simulink model "ACC_2022b"  (R2022b)
settings: Solver=VariableStepAuto  StartTime=0.0  StopTime=inf  RelTol=1e-3
values from neighbouring files (symbols this model uses):
  b = 50    [ACC_code.m]
  D_default = 10    [ACC_code.m]
  m = 1000    [ACC_code.m]
undefined symbols (not defined in the file or in its folder): Ego_acceleration_max, Ego_acceleration_min, Ego_position_initial, Ego_velocity_initial_kmh, h, km, Kverr_gain, Kvx_gain, Kxerr_gain, Lead_position_initial, Lead_velocity_initial_kmh, s
libraries: aerolibconvert2 x6
settings Model: PacingRate=2  Creator=Leo  LastModifiedBy=Usuario
settings OptimizationCC: BlockReduction=off  DefaultParameterBehavior=Inlined  BufferReuse=off  ReuseModelBlockBuffer=on

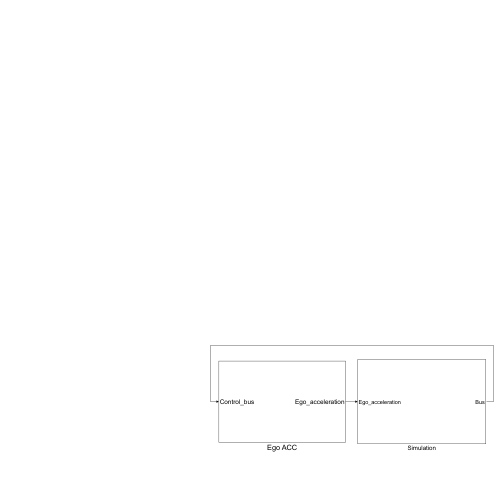
[thumbnail: Simulink's stored preview of the top-level diagram]
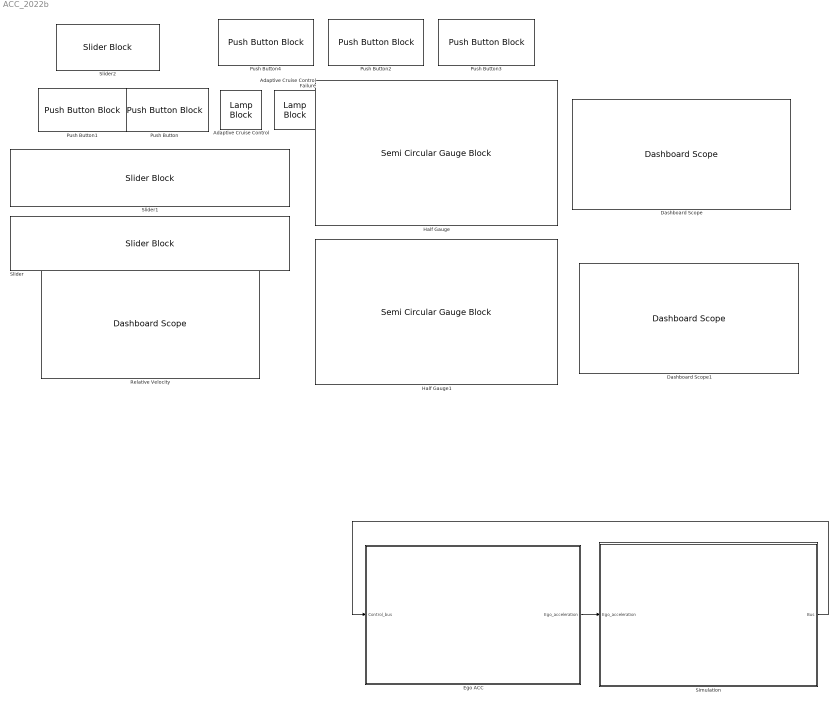
== system ACC_2022b ==
  Adaptive Cruise Control : LampBlock  LabelPosition=Hide  Icon=AdaptiveCruiseControl
  Adaptive Cruise Control Failure : LampBlock  LabelPosition=Hide  Icon=AdaptiveCruiseControlFailure
  Dashboard Scope : DashboardScope
  Dashboard Scope1 : DashboardScope
  Ego ACC : Subsystem
  Half Gauge : SemiCircularGaugeBlock  ScaleMax=220  TickInterval=20
  Half Gauge1 : SemiCircularGaugeBlock  ScaleMax=220  TickInterval=20
  Push Button : PushButtonBlock  ButtonText=ACC  OffValue=0.000000
  Push Button1 : PushButtonBlock  ButtonText=Rain  OffValue=0.000000
  Push Button2 : PushButtonBlock  ButtonText=Gas  ButtonType=Latch
  Push Button3 : PushButtonBlock  ButtonText=Brake  ButtonType=Latch
  Push Button4 : PushButtonBlock  ButtonText=Fault  ButtonType=Latch  OffValue=0.000000
  Relative Velocity : DashboardScope
  Simulation : Subsystem
  Slider : SliderBlock  ScaleMax=220  TickInterval=50
  Slider1 : SliderBlock  ScaleMin=40  ScaleMax=220  TickInterval=50
  Slider2 : SliderBlock  ScaleMin=1  ScaleMax=3  TickInterval=0.5
  wires:
  Ego ACC/1(Ego_acceleration) -> Simulation/1(Ego_acceleration)
  Simulation/1(Bus) -> Ego ACC/1(Control_bus)

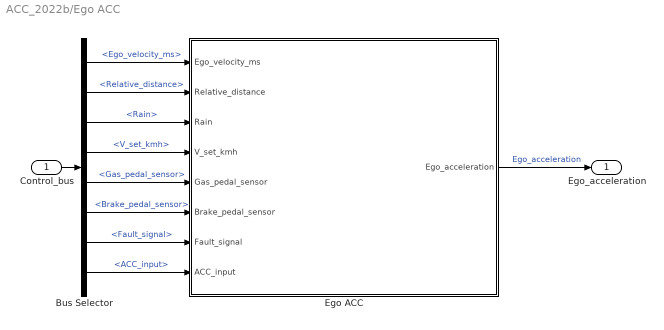
== system ACC_2022b/Ego ACC ==
  Control_bus : Inport
  Bus Selector : BusSelector  OutputSignals=Ego_velocity_ms,Relative_distance,Rain,V_set_kmh,Gas_pedal_sensor,Brake_pedal_sensor,Fault_signal,ACC_input
  Ego ACC : Subsystem
  Ego_acceleration : Outport
  wires:
  Control_bus/1 -> Bus Selector/1
  Ego ACC/1(Ego_acceleration) -> Ego_acceleration/1  "Ego_acceleration"
  Bus Selector/1 -> Ego ACC/1(Ego_velocity_ms)  "<Ego_velocity_ms>"
  Bus Selector/2 -> Ego ACC/2(Relative_distance)  "<Relative_distance>"
  Bus Selector/3 -> Ego ACC/3(Rain)  "<Rain>"
  Bus Selector/4 -> Ego ACC/4(V_set_kmh)  "<V_set_kmh>"
  Bus Selector/5 -> Ego ACC/5(Gas_pedal_sensor)  "<Gas_pedal_sensor>"
  Bus Selector/6 -> Ego ACC/6(Brake_pedal_sensor)  "<Brake_pedal_sensor>"
  Bus Selector/7 -> Ego ACC/7(Fault_signal)  "<Fault_signal>"
  Bus Selector/8 -> Ego ACC/8(ACC_input)  "<ACC_input>"

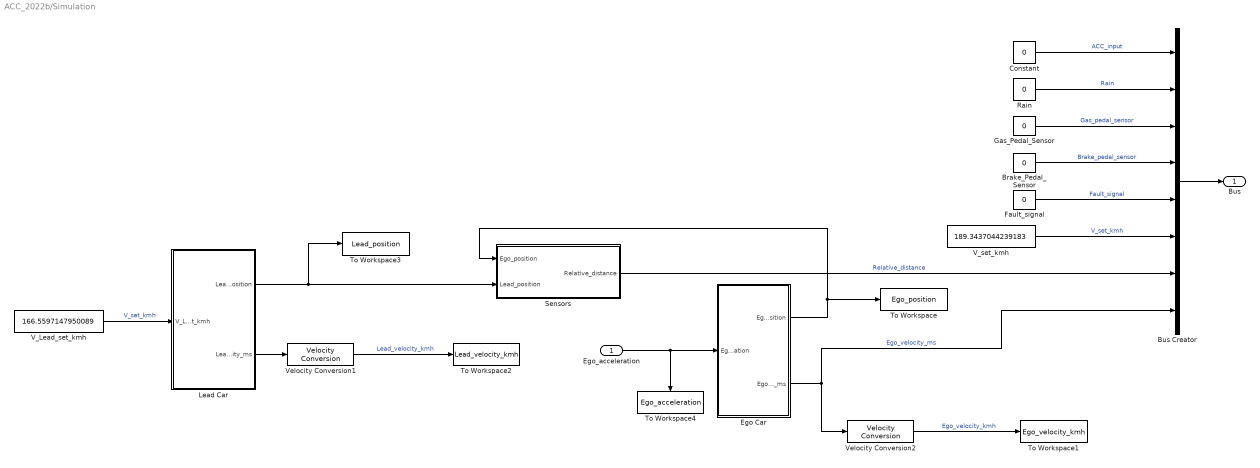
== system ACC_2022b/Simulation ==
  Ego_acceleration : Inport
  Brake_Pedal_Sensor : Constant  Value=0  SampleTime=-1
  Bus Creator : BusCreator  Inputs=8
  Constant : Constant  Value=0
  Ego Car : Subsystem
  Fault_signal : Constant  Value=0  SampleTime=-1
  Gas_Pedal_Sensor : Constant  Value=0  SampleTime=-1
  Lead Car : Subsystem
  Rain : Constant  Value=0
  Sensors : Subsystem
  To Workspace : ToWorkspace  VariableName=Ego_position  SaveFormat=Timeseries  SampleTime=-1
  To Workspace1 : ToWorkspace  VariableName=Ego_velocity_kmh  SaveFormat=Timeseries  SampleTime=-1
  To Workspace2 : ToWorkspace  VariableName=Lead_velocity_kmh  SaveFormat=Timeseries  SampleTime=-1
  To Workspace3 : ToWorkspace  VariableName=Lead_position  SaveFormat=Timeseries  SampleTime=-1
  To Workspace4 : ToWorkspace  VariableName=Ego_acceleration  SaveFormat=Timeseries  SampleTime=-1
  V_Lead_set_kmh : Constant  Value=166.5597147950089  SampleTime=-1
  V_set_kmh : Constant  Value=189.3437044239183  SampleTime=-1
  Velocity Conversion1 : aerolibconvert2/Velocity Conversion  IU=m/s  OU=km/h
  Velocity Conversion2 : aerolibconvert2/Velocity Conversion  IU=m/s  OU=km/h
  Bus : Outport
  wires:
  Constant/1 -> Bus Creator/1  "ACC_input"
  Lead Car/1(Lead_position) -> To Workspace3/1, Sensors/2(Lead_position)
  Fault_signal/1 -> Bus Creator/5  "Fault_signal"
  Sensors/1(Relative_distance) -> Bus Creator/7  "Relative_distance"
  Rain/1 -> Bus Creator/2  "Rain"
  Gas_Pedal_Sensor/1 -> Bus Creator/3  "Gas_pedal_sensor"
  Ego Car/1(Ego_position) -> To Workspace/1, Sensors/1(Ego_position)
  Brake_Pedal_Sensor/1 -> Bus Creator/4  "Brake_pedal_sensor"
  V_set_kmh/1 -> Bus Creator/6  "V_set_kmh"
  Ego Car/2(Ego_velocity_ms) -> Velocity Conversion2/1, Bus Creator/8  "Ego_velocity_ms"
  Bus Creator/1 -> Bus/1
  Ego_acceleration/1 -> To Workspace4/1, Ego Car/1(Ego_acceleration)
  Velocity Conversion1/1 -> To Workspace2/1  "Lead_velocity_kmh"
  Velocity Conversion2/1 -> To Workspace1/1  "Ego_velocity_kmh"
  Lead Car/2(Lead_velocity_ms) -> Velocity Conversion1/1
  V_Lead_set_kmh/1 -> Lead Car/1(V_Lead_Set_kmh)  "V_set_kmh"

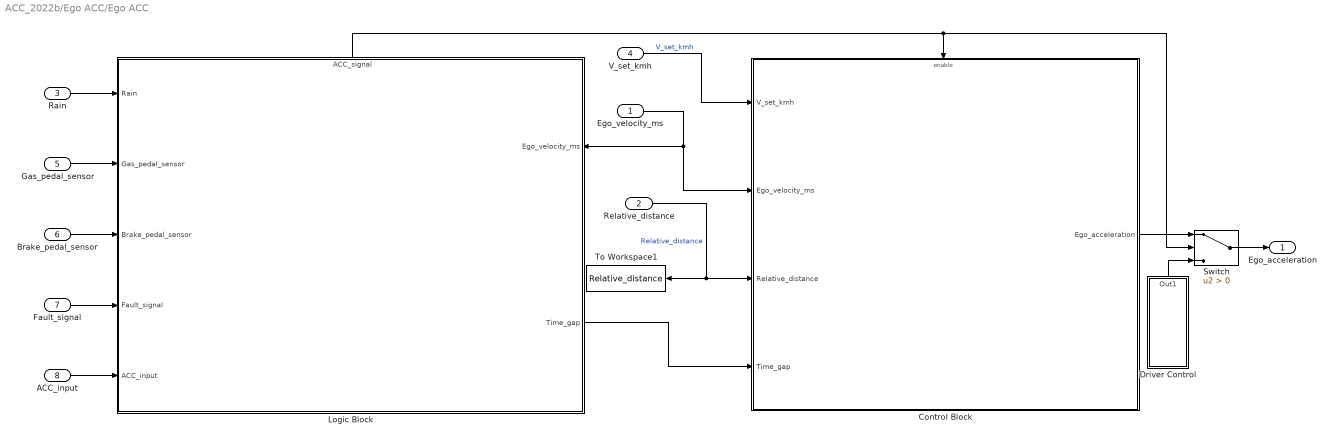
== system ACC_2022b/Ego ACC/Ego ACC ==
  Ego_velocity_ms : Inport
  Relative_distance : Inport  Port=2
  Rain : Inport  Port=3
  V_set_kmh : Inport  Port=4
  Gas_pedal_sensor : Inport  Port=5
  Brake_pedal_sensor : Inport  Port=6
  Fault_signal : Inport  Port=7
  ACC_input : Inport  Port=8
  Control Block : Subsystem
  Driver Control : Subsystem
  Logic Block : Subsystem
      settings: PortSchema="{\"entries\":[{\"content\":{\"sides\":[{\"content\":{\"connectorIds\":[\"In1\",\"In2\",\"In3\",\"In4\",\"In5\"]},\"type\":\"ConnectorPlacement.EquallySpacedRectSide\",\"uuid\":\"6fa6196d-b048-4bc1-969a-f090033d4757\"},{\"content\":{\"connectorIds\":[\"In6\",\"Out1\"],\"side\":\"RIGHT\"},\"type\":\"ConnectorPlacement.EquallySpacedRectSide\",\"uuid\":\"e0f255d9-e478-45fe-ae77-17524099c0e9\"},{\"content\":{\"connectorIds\":[\"Out2\"],\"side\":\"TOP\"},\"type\":\"ConnectorPlacement.EquallySpacedRectSide\",\"uuid\":\"d378020a-93ed-4543-a71a-2f5d1fd34348\"}]},\"type\":\"ConnectorPlacement.EquallySpacedConnector\",\"uuid\":\"05add8da-79bb-421f-8702-7cb44b699c82\"}],\"packageUris\":[\"http://schema.mathworks.com/mf0/Connector/R2020b\"],\"version\":\"1.0\"}"
  Switch : Switch  Criteria=u2 > Threshold  SaturateOnIntegerOverflow=off  InputSameDT=off
  To Workspace1 : ToWorkspace  VariableName=Relative_distance  SaveFormat=Timeseries  SampleTime=-1
  Ego_acceleration : Outport  VectorParamsAs1DForOutWhenUnconnected=off
  wires:
  V_set_kmh/1 -> Control Block/1(V_set_kmh)  "V_set_kmh"
  Ego_velocity_ms/1 -> Control Block/2(Ego_velocity_ms), Logic Block/6(Ego_velocity_ms)
  Relative_distance/1 -> To Workspace1/1, Control Block/3(Relative_distance)  "Relative_distance"
  Control Block/1(Ego_acceleration) -> Switch/1
  Rain/1 -> Logic Block/1(Rain)
  Gas_pedal_sensor/1 -> Logic Block/2(Gas_pedal_sensor)
  Brake_pedal_sensor/1 -> Logic Block/3(Brake_pedal_sensor)
  Fault_signal/1 -> Logic Block/4(Fault_signal)
  ACC_input/1 -> Logic Block/5(ACC_input)
  Logic Block/2(ACC_signal) -> Control Block/Enable, Switch/2
  Logic Block/1(Time_gap) -> Control Block/4(Time_gap)
  Switch/1 -> Ego_acceleration/1
  Driver Control/1(Out1) -> Switch/3

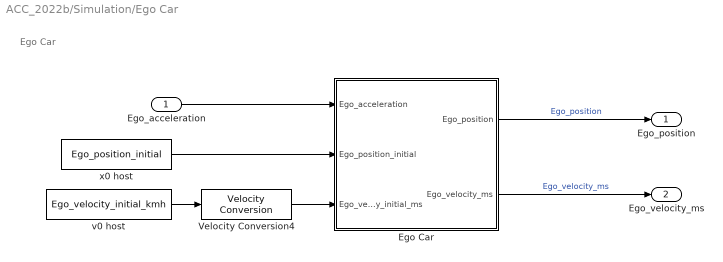
== system ACC_2022b/Simulation/Ego Car ==
  note: Ego Car
  Ego_acceleration : Inport
  Ego Car : Subsystem
  Velocity Conversion4 : aerolibconvert2/Velocity Conversion  IU=km/h  OU=m/s
  v0 host : Constant  Value=Ego_velocity_initial_kmh  SampleTime=-1
  x0 host : Constant  Value=Ego_position_initial  SampleTime=-1
  Ego_position : Outport
  Ego_velocity_ms : Outport  Port=2
  wires:
  Velocity Conversion4/1 -> Ego Car/3(Ego_velocity_initial_ms)
  x0 host/1 -> Ego Car/2(Ego_position_initial)
  v0 host/1 -> Velocity Conversion4/1
  Ego Car/1(Ego_position) -> Ego_position/1  "Ego_position"
  Ego Car/2(Ego_velocity_ms) -> Ego_velocity_ms/1  "Ego_velocity_ms"
  Ego_acceleration/1 -> Ego Car/1(Ego_acceleration)

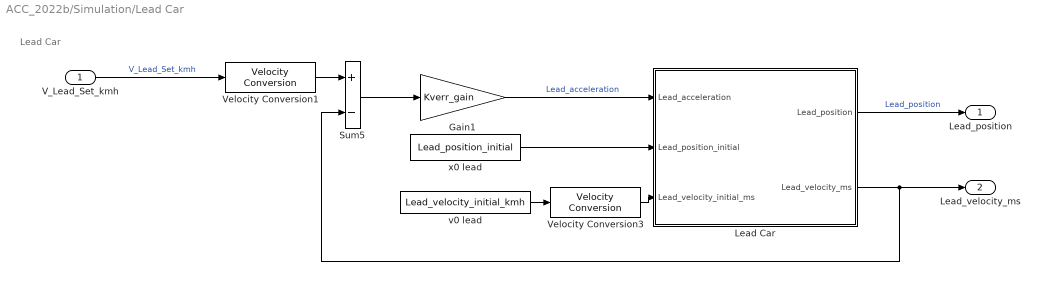
== system ACC_2022b/Simulation/Lead Car ==
  note: Lead Car
  V_Lead_Set_kmh : Inport
  Gain1 : Gain  Gain=Kverr_gain
  Lead Car : Subsystem
  Sum5 : Sum  Inputs=+-
  Velocity Conversion1 : aerolibconvert2/Velocity Conversion  IU=km/h  OU=m/s
  Velocity Conversion3 : aerolibconvert2/Velocity Conversion  IU=km/h  OU=m/s
  v0 lead : Constant  Value=Lead_velocity_initial_kmh  SampleTime=-1
  x0 lead : Constant  Value=Lead_position_initial  SampleTime=-1
  Lead_position : Outport
  Lead_velocity_ms : Outport  Port=2
  wires:
  x0 lead/1 -> Lead Car/2(Lead_position_initial)
  Lead Car/2(Lead_velocity_ms) -> Sum5/2, Lead_velocity_ms/1
  Velocity Conversion3/1 -> Lead Car/3(Lead_velocity_initial_ms)
  Lead Car/1(Lead_position) -> Lead_position/1  "Lead_position"
  Gain1/1 -> Lead Car/1(Lead_acceleration)  "Lead_acceleration"
  v0 lead/1 -> Velocity Conversion3/1
  Velocity Conversion1/1 -> Sum5/1
  V_Lead_Set_kmh/1 -> Velocity Conversion1/1  "V_Lead_Set_kmh"
  Sum5/1 -> Gain1/1

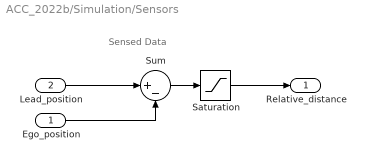
== system ACC_2022b/Simulation/Sensors ==
  note: Sensed Data
  Ego_position : Inport
  Lead_position : Inport  Port=2
  Saturation : Saturate  UpperLimit=200  LowerLimit=0
  Sum : Sum  Inputs=|+-
  Relative_distance : Outport
  wires:
  Sum/1 -> Saturation/1
  Ego_position/1 -> Sum/2
  Saturation/1 -> Relative_distance/1
  Lead_position/1 -> Sum/1

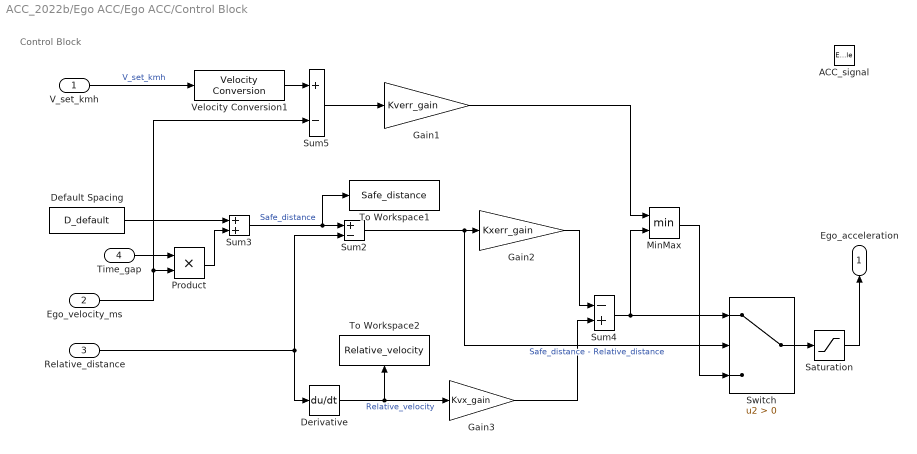
== system ACC_2022b/Ego ACC/Ego ACC/Control Block ==
  note: Control Block
  V_set_kmh : Inport
  Ego_velocity_ms : Inport  Port=2
  Relative_distance : Inport  Port=3
  Time_gap : Inport  Port=4
  ACC_signal : EnablePort  StatesWhenEnabling=reset
  Default Spacing : Constant  Value=D_default  SampleTime=-1
  Derivative : Derivative
  Gain1 : Gain  Gain=Kverr_gain
  Gain2 : Gain  Gain=Kxerr_gain
  Gain3 : Gain  Gain=Kvx_gain
  MinMax : MinMax  Inputs=2
  Product : Product
  Saturation : Saturate  UpperLimit=Ego_acceleration_max  LowerLimit=Ego_acceleration_min
  Sum2 : Sum  Inputs=+-
  Sum3 : Sum
  Sum4 : Sum  Inputs=-+
  Sum5 : Sum  Inputs=+-
  Switch : Switch  Criteria=u2 > Threshold  SaturateOnIntegerOverflow=off  InputSameDT=off
  To Workspace1 : ToWorkspace  VariableName=Safe_distance  SaveFormat=Timeseries  SampleTime=-1
  To Workspace2 : ToWorkspace  VariableName=Relative_velocity  SaveFormat=Timeseries  SampleTime=-1
  Velocity Conversion1 : aerolibconvert2/Velocity Conversion  IU=km/h  OU=m/s
  Ego_acceleration : Outport  InitialOutput=0  VectorParamsAs1DForOutWhenUnconnected=off
  wires:
  Sum5/1 -> Gain1/1
  Default Spacing/1 -> Sum3/1
  Relative_distance/1 -> Derivative/1, Sum2/2
  Sum2/1 -> Switch/2, Gain2/1  "Safe_distance - Relative_distance"
  Sum4/1 -> Switch/1, MinMax/2
  Switch/1 -> Saturation/1
  MinMax/1 -> Switch/3
  Product/1 -> Sum3/2
  Sum3/1 -> To Workspace1/1, Sum2/1  "Safe_distance"
  Gain1/1 -> MinMax/1
  Gain2/1 -> Sum4/1
  Ego_velocity_ms/1 -> Product/2, Sum5/2
  V_set_kmh/1 -> Velocity Conversion1/1  "V_set_kmh"
  Saturation/1 -> Ego_acceleration/1
  Velocity Conversion1/1 -> Sum5/1
  Time_gap/1 -> Product/1
  Gain3/1 -> Sum4/2
  Derivative/1 -> Gain3/1, To Workspace2/1  "Relative_velocity"

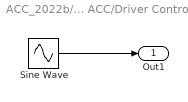
== system ACC_2022b/Ego ACC/Ego ACC/Driver Control ==
  Sine Wave : Sin  Amplitude=0.1  Frequency=0.1
  Out1 : Outport
  wires:
  Sine Wave/1 -> Out1/1

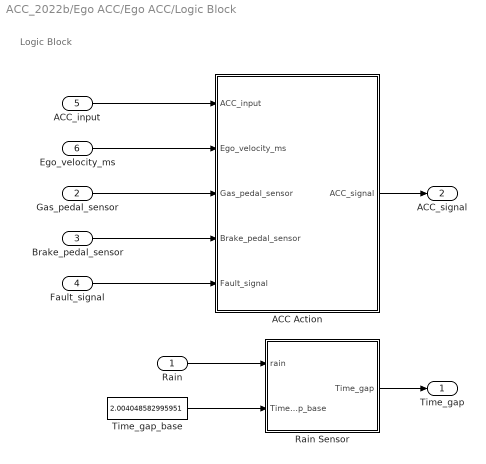
== system ACC_2022b/Ego ACC/Ego ACC/Logic Block ==
  note: Logic Block
  Rain : Inport
  Gas_pedal_sensor : Inport  Port=2
  Brake_pedal_sensor : Inport  Port=3
  Fault_signal : Inport  Port=4
  ACC_input : Inport  Port=5
  Ego_velocity_ms : Inport  Port=6
  ACC Action : Stateflow chart  TreatAsAtomicUnit=on
  Rain Sensor : Stateflow chart  TreatAsAtomicUnit=on
  Time_gap_base : Constant  Value=2.004048582995951  SampleTime=-1
  Time_gap : Outport
  ACC_signal : Outport  Port=2
  wires:
  ACC_input/1 -> ACC Action/1(ACC_input)
  Rain/1 -> Rain Sensor/1(rain)
  ACC Action/1(ACC_signal) -> ACC_signal/1
  Rain Sensor/1(Time_gap) -> Time_gap/1
  Time_gap_base/1 -> Rain Sensor/2(Time_gap_base)
  Ego_velocity_ms/1 -> ACC Action/2(Ego_velocity_ms)
  Gas_pedal_sensor/1 -> ACC Action/3(Gas_pedal_sensor)
  Brake_pedal_sensor/1 -> ACC Action/4(Brake_pedal_sensor)
  Fault_signal/1 -> ACC Action/5(Fault_signal)

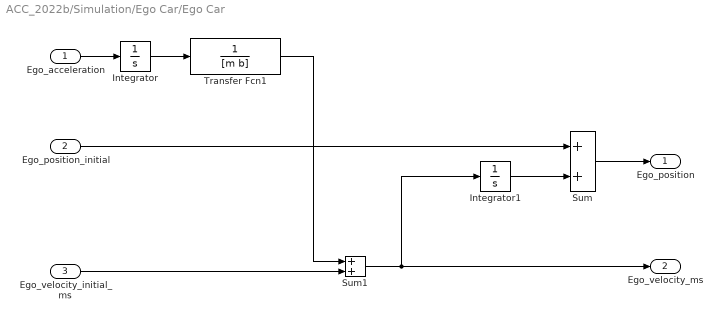
== system ACC_2022b/Simulation/Ego Car/Ego Car ==
  Ego_acceleration : Inport
  Ego_position_initial : Inport  Port=2
  Ego_velocity_initial_ms : Inport  Port=3
  Integrator : Integrator
  Integrator1 : Integrator
  Sum : Sum
  Sum1 : Sum
  Transfer Fcn1 : TransferFcn  Denominator=[m b]
  Ego_position : Outport  VectorParamsAs1DForOutWhenUnconnected=off
  Ego_velocity_ms : Outport  Port=2  VectorParamsAs1DForOutWhenUnconnected=off
  wires:
  Sum1/1 -> Integrator1/1, Ego_velocity_ms/1
  Ego_velocity_initial_ms/1 -> Sum1/2
  Sum/1 -> Ego_position/1
  Transfer Fcn1/1 -> Sum1/1
  Ego_acceleration/1 -> Integrator/1
  Ego_position_initial/1 -> Sum/1
  Integrator1/1 -> Sum/2
  Integrator/1 -> Transfer Fcn1/1

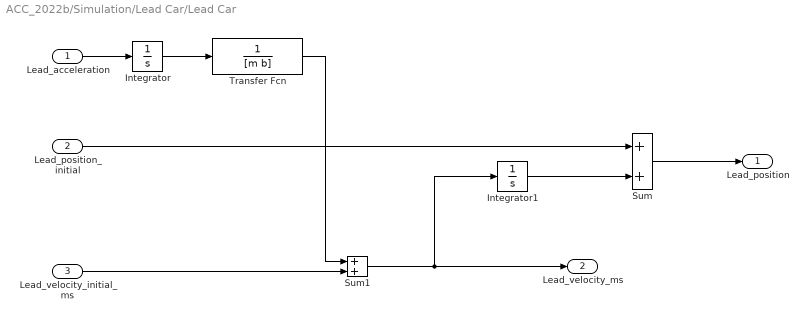
== system ACC_2022b/Simulation/Lead Car/Lead Car ==
  Lead_acceleration : Inport
  Lead_position_initial : Inport  Port=2
  Lead_velocity_initial_ms : Inport  Port=3
  Integrator : Integrator
  Integrator1 : Integrator
  Sum : Sum
  Sum1 : Sum
  Transfer Fcn : TransferFcn  Denominator=[m b]
  Lead_position : Outport  VectorParamsAs1DForOutWhenUnconnected=off
  Lead_velocity_ms : Outport  Port=2  VectorParamsAs1DForOutWhenUnconnected=off
  wires:
  Transfer Fcn/1 -> Sum1/1
  Lead_velocity_initial_ms/1 -> Sum1/2
  Sum/1 -> Lead_position/1
  Lead_acceleration/1 -> Integrator/1
  Sum1/1 -> Integrator1/1, Lead_velocity_ms/1
  Lead_position_initial/1 -> Sum/1
  Integrator1/1 -> Sum/2
  Integrator/1 -> Transfer Fcn/1

== stateflow chart ACC_2022b/Ego ACC/Ego ACC/Logic Block/ACC Action ==
  state Operational
    state Init
      entry:
      ACC_signal = 0;
      Ego_velocity_local = Ego_velocity_ms;
    state Otherstage
      entry:
      ACC_signal = 0;
      during:
      Ego_velocity_local = Ego_velocity_ms;
    state Nextstage
      entry:
      ACC_signal = 0;
      during:
      Ego_velocity_local = Ego_velocity_ms;
    state Finalstage
      entry:
      ACC_signal = 1;
      during:
      Ego_velocity_local = Ego_velocity_ms;
    (default) -> Init
    Init -> Nextstage : [Ego_velocity_local>=11]
    Otherstage -> Nextstage : [Ego_velocity_local >= 11]
    Nextstage -> Otherstage [order 2] : [Ego_velocity_local < 11]
    Finalstage -> Otherstage : [hasChangedFrom(ACC_input,0) || Gas_pedal_sensor == 1 || Brake_pedal_sensor == 1]
    Nextstage -> Finalstage [order 1] : [hasChangedFrom(ACC_input,0) && Gas_pedal_sensor == 0 && Brake_pedal_sensor == 0]
  state Disabled
    entry:
    ACC_signal = 0;
  (default) -> Operational
  Disabled -> Operational : [Fault_signal == 0]
  Operational -> Disabled : [Fault_signal == 1]
  data: ACC_signal output; ACC_input input; Ego_velocity_ms input; Gas_pedal_sensor input; Ego_velocity_local local; Brake_pedal_sensor input; Fault_signal input

== stateflow chart ACC_2022b/Ego ACC/Ego ACC/Logic Block/Rain Sensor ==
  state no_rain
    entry:
    Time_gap = Time_gap_base;
  state rain
    entry:
    Time_gap = 2*Time_gap_base;
  (default) -> no_rain
  no_rain -> rain : [rain == 1]
  rain -> no_rain : [rain == 0]
  data: rain input; Time_gap output; Time_gap_base input
